simulink model "exampleRadiatorBasic"  (Simulink 7.6)
settings: Solver=ode45  StartTime=0.0  StopTime=8*3600  RelTol=1e-3
undefined symbols (not defined in the file): A, B, C, Dd
libraries: carnot x6
settings Model: Creator=drhf  LastModifiedBy=drhf

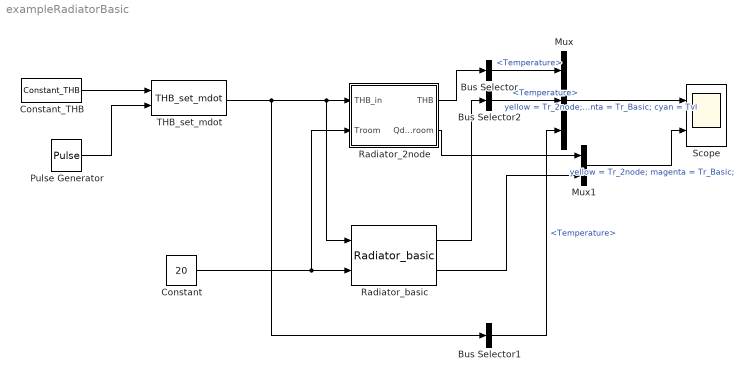
== system exampleRadiatorBasic ==
  Bus Selector : BusSelector  OutputSignals=Temperature
  Bus Selector1 : BusSelector  OutputSignals=Temperature
  Bus Selector2 : BusSelector  OutputSignals=Temperature
  Constant : Constant  Value=20
  Constant_THB : carnot/Source/Simple/Constant_THB  SystemSampleTime=-1  t=75  mdot=0*100/3600  p=1e5  mID=No Pressure Drop  fluid=Water  mix=0  dia=0.02  hgt=0
  Mux : Mux  Inputs=3
  Mux1 : Mux  Inputs=2
  Pulse Generator : DiscretePulseGenerator  PulseType=Time based  Amplitude=100/3600  Period=4*3600  PulseWidth=50
  Radiator_2node : Subsystem  mask(basic radiator){pnom=1200, dtnom=50, expo=1.3, mcp=4182*1, lin=100, qua=100}
      mask prompts: pnom "Qdot_nom: nominal power per in W"; dtnom "Tdiff_nom: nominal temperature difference in K"; expo "radiator exponent (> 0)"; mcp "mass * capacity per unit in J/K"; lin "linear pressure drop"; qua "quadratic pressure drop"
      mask help:
      | The block calculates the heat transfer of a radiator to a room according to the EN 442 equation.
      | A quadratic pressure drop is applied to the fluid flow.
  Radiator_basic : carnot/Basic/Thermal_Models/Radiator_basic  SystemSampleTime=-1  pnomEN=1000  dtnomEN=50  expo=1.3  mcp=4182*1
  Scope : Scope  NumInputPorts=2
      settings: YMin=-5~-5  YMax=5~5
  THB_set_mdot : carnot/Source/Simple/THB_set_mdot  SystemSampleTime=-1
  wires:
  Constant/1 -> Radiator_2node/2(Troom), Radiator_basic/2
  Constant_THB/1 -> THB_set_mdot/1
  THB_set_mdot/1 -> Radiator_2node/1(THB_in), Radiator_basic/1, Bus Selector1/1
  Pulse Generator/1 -> THB_set_mdot/2
  Radiator_2node/1(THB) -> Bus Selector/1
  Bus Selector/1 -> Mux/1  "<Temperature>"
  Mux/1 -> Scope/1  "yellow = Tr_2node; magenta = Tr_Basic; cyan = Tvl"
  Radiator_2node/2(Qdot2room) -> Mux1/1
  Mux1/1 -> Scope/2  "yellow = Tr_2node; magenta = Tr_Basic;"
  Radiator_basic/2 -> Mux1/2
  Radiator_basic/1 -> Bus Selector2/1
  Bus Selector2/1 -> Mux/2  "<Temperature>"
  Bus Selector1/1 -> Mux/3  "<Temperature>"

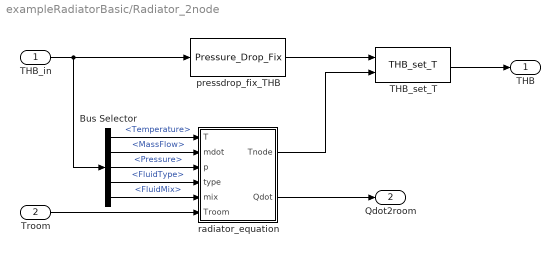
== system exampleRadiatorBasic/Radiator_2node ==
  THB_in : Inport
  Troom : Inport  Port=2
  Bus Selector : BusSelector  OutputSignals=Temperature,MassFlow,Pressure,FluidType,FluidMix
  THB_set_T : carnot/Source/Simple/THB_set_T  SystemSampleTime=-1
  pressdrop_fix_THB : carnot/Basic/Pressure_Drop/Pressure_Drop_Fix  SystemSampleTime=-1  con=0  lin=lin  qua=qua
  radiator_equation : Subsystem  mask(radiator equation){pnom=pnom, dtnom=dtnom, expo=expo, mcap=mcp}
      mask prompts: pnom "Qdot_nom: nominal power per in W"; dtnom "Tdiff_nom: nominal temperature difference in K"; expo "radiator exponent (> 0)"; mcap "mass * capacity per unit in J/K"
      mask help:
      | The block calculates the heat transfer of a radiator to a room according to the EN 442 equation:
      | Qdot = Qdot_nom * (Tdiff/Tdiff_nom)^exponent
      | The thermal capacity of the radiator is modeled by a 1-node capacity.
      | mcp*dT/dt = mdot*cp*(Tin-Tnode)-Qdot
  THB : Outport
  Qdot2room : Outport  Port=2
  wires:
  radiator_equation/2(Qdot) -> Qdot2room/1
  Troom/1 -> radiator_equation/6(Troom)
  radiator_equation/1(Tnode) -> THB_set_T/2
  THB_in/1 -> Bus Selector/1, pressdrop_fix_THB/1
  pressdrop_fix_THB/1 -> THB_set_T/1
  THB_set_T/1 -> THB/1
  Bus Selector/3 -> radiator_equation/3(p)  "<Pressure>"
  Bus Selector/4 -> radiator_equation/4(type)  "<FluidType>"
  Bus Selector/5 -> radiator_equation/5(mix)  "<FluidMix>"
  Bus Selector/2 -> radiator_equation/2(mdot)  "<MassFlow>"
  Bus Selector/1 -> radiator_equation/1(T)  "<Temperature>"

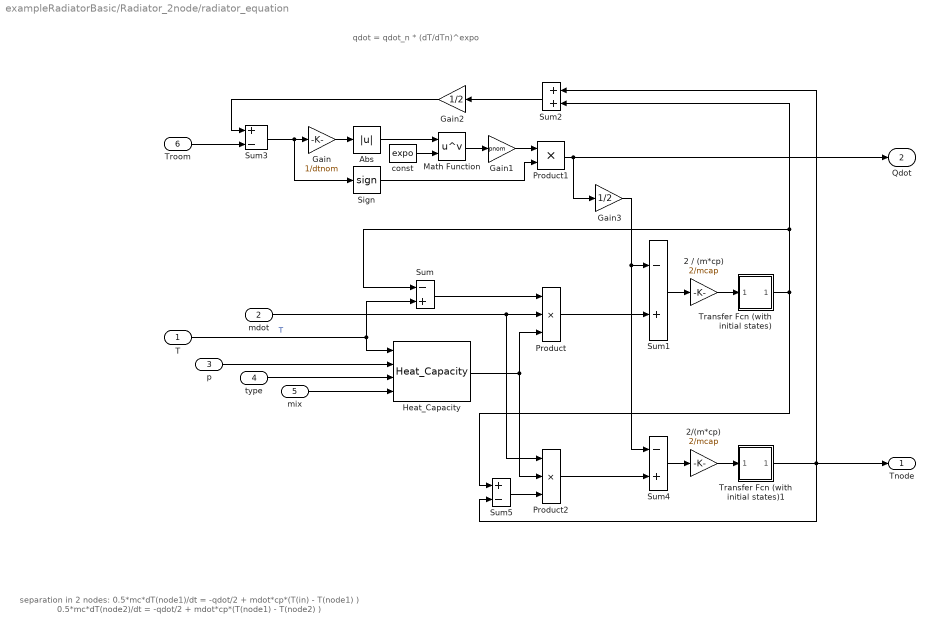
== system exampleRadiatorBasic/Radiator_2node/radiator_equation ==
  note: separation in 2 nodes:
      | 0.5*mc*dT(node1)/dt = -qdot/2 + mdot*cp*(T(in) - T(node1) )
      | 0.5*mc*dT(node2)/dt = -qdot/2 + mdot*cp*(T(node1) - T(node2) )
  note: qdot = qdot_n * (dT/dTn)^expo
  T : Inport
  mdot : Inport  Port=2
  p : Inport  Port=3
  type : Inport  Port=4
  mix : Inport  Port=5
  Troom : Inport  Port=6
  2 / (m*cp) : Gain  Gain=2/mcap  SaturateOnIntegerOverflow=on  OutDataTypeStr=Inherit: Same as input  ParamDataTypeStr=Inherit: Same as input
  2/(m*cp) : Gain  Gain=2/mcap  SaturateOnIntegerOverflow=on  OutDataTypeStr=Inherit: Same as input  ParamDataTypeStr=Inherit: Same as input
  Abs : Abs  SaturateOnIntegerOverflow=on
  Gain : Gain  Gain=1/dtnom  SaturateOnIntegerOverflow=on  OutDataTypeStr=Inherit: Same as input  ParamDataTypeStr=Inherit: Same as input
  Gain1 : Gain  Gain=pnom  SaturateOnIntegerOverflow=on  OutDataTypeStr=Inherit: Same as input  ParamDataTypeStr=Inherit: Same as input
  Gain2 : Gain  Gain=1/2  SaturateOnIntegerOverflow=on  OutDataTypeStr=Inherit: Same as input  ParamDataTypeStr=Inherit: Same as input
  Gain3 : Gain  Gain=1/2  SaturateOnIntegerOverflow=on  OutDataTypeStr=Inherit: Same as input  ParamDataTypeStr=Inherit: Same as input
  Heat_Capacity : carnot/Basic/Material_Properties/Heat_Capacity  SystemSampleTime=-1  VariantObject=CarlibClassic  INPUTARGUMENTS=state variables (classic)  DEBUGLEVEL=DEBUGLEVEL  MAXTOTALWARNINGS=inf  MAXCONSECUTIVEWARNINGS=inf  WRITETOFILE=0  FILENAME='errors.txt'
  Math Function : Math  Operator=pow  SaturateOnIntegerOverflow=on
  Product : Product  Inputs=3  SaturateOnIntegerOverflow=on  InputSameDT=on  OutDataTypeStr=Inherit: Same as first input
  Product1 : Product  SaturateOnIntegerOverflow=on  InputSameDT=on  OutDataTypeStr=Inherit: Same as first input
  Product2 : Product  Inputs=3  SaturateOnIntegerOverflow=on  InputSameDT=on  OutDataTypeStr=Inherit: Same as first input
  Sign : Signum
  Sum : Sum  Inputs=-+  SaturateOnIntegerOverflow=on  InputSameDT=on  OutDataTypeStr=Inherit: Same as first input
  Sum1 : Sum  Inputs=-+  SaturateOnIntegerOverflow=on  InputSameDT=on  OutDataTypeStr=Inherit: Same as first input
  Sum2 : Sum  Inputs=2  SaturateOnIntegerOverflow=on  InputSameDT=on  OutDataTypeStr=Inherit: Same as first input
  Sum3 : Sum  Inputs=+-  SaturateOnIntegerOverflow=on  InputSameDT=on  OutDataTypeStr=Inherit: Same as first input
  Sum4 : Sum  Inputs=-+  SaturateOnIntegerOverflow=on  InputSameDT=on  OutDataTypeStr=Inherit: Same as first input
  Sum5 : Sum  Inputs=+-  SaturateOnIntegerOverflow=on  InputSameDT=on  OutDataTypeStr=Inherit: Same as first input
  Transfer Fcn (with initial states) : Subsystem  mask(Transfer Function with Initial States){N=[1], D=[1  0], X0=20}
      mask prompts: N "Numerator:"; D "Denominator:"; X0 "Initial conditions:"
      mask help: Vector expressions for numerator, and denominator. Coefficients are in descending powers of s.
      mask init:
      | [A,B,C,Dd]=tf2ss(N,D);if (isempty(X0));[m,n]=size(A);X0=zeros(1,m); end;
      mask Help: Specify the initial states for the transfer function.  The state ordering is determined by the m-file tf2ss.  There is no unique mapping of the states in a transfer function to states in a state-space representation.  However, tf2ss will consistently use the same mapping for a given transfer function.
      mask Display: dpoly(N,D,'s')
  Transfer Fcn (with initial states)1 : Subsystem  mask(Transfer Function with Initial States){N=[1], D=[1  0], X0=20}
      mask prompts: N "Numerator:"; D "Denominator:"; X0 "Initial conditions:"
      mask help: Vector expressions for numerator, and denominator. Coefficients are in descending powers of s.
      mask init:
      | [A,B,C,Dd]=tf2ss(N,D);if (isempty(X0));[m,n]=size(A);X0=zeros(1,m); end;
      mask Help: Specify the initial states for the transfer function.  The state ordering is determined by the m-file tf2ss.  There is no unique mapping of the states in a transfer function to states in a state-space representation.  However, tf2ss will consistently use the same mapping for a given transfer function.
      mask Display: dpoly(N,D,'s')
  const : Constant  Value=expo
  Tnode : Outport
  Qdot : Outport  Port=2
  wires:
  Transfer Fcn (with initial states)/1(Out1) -> Sum2/2, Sum/1, Sum5/1
  2 / (m*cp)/1 -> Transfer Fcn (with initial states)/1(In1)
  Sum1/1 -> 2 / (m*cp)/1
  Product/1 -> Sum1/2
  Heat_Capacity/1 -> Product/3, Product2/2
  T/1 -> Sum/2, Heat_Capacity/1  "T"
  mdot/1 -> Product/2, Product2/1
  Sum/1 -> Product/1
  p/1 -> Heat_Capacity/2
  type/1 -> Heat_Capacity/3
  mix/1 -> Heat_Capacity/4
  Product1/1 -> Qdot/1, Gain3/1
  const/1 -> Math Function/2
  Math Function/1 -> Gain1/1
  Gain/1 -> Abs/1
  Abs/1 -> Math Function/1
  Gain1/1 -> Product1/1
  Sum3/1 -> Gain/1, Sign/1
  Sign/1 -> Product1/2
  Troom/1 -> Sum3/2
  Gain2/1 -> Sum3/1
  Sum2/1 -> Gain2/1
  2/(m*cp)/1 -> Transfer Fcn (with initial states)1/1(In1)
  Sum4/1 -> 2/(m*cp)/1
  Gain3/1 -> Sum1/1, Sum4/1
  Sum5/1 -> Product2/3
  Transfer Fcn (with initial states)1/1(Out1) -> Sum5/2, Tnode/1, Sum2/1
  Product2/1 -> Sum4/2

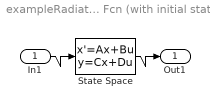
== system exampleRadiatorBasic/Radiator_2node/radiator_equation/Transfer Fcn (with initial states) ==
  In1 : Inport
  State Space : StateSpace  A=A  B=B  C=C  D=Dd  X0=X0
  Out1 : Outport  InitialOutput=0
  wires:
  In1/1 -> State Space/1
  State Space/1 -> Out1/1

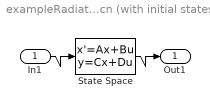
== system exampleRadiatorBasic/Radiator_2node/radiator_equation/Transfer Fcn (with initial states)1 ==
  In1 : Inport
  State Space : StateSpace  A=A  B=B  C=C  D=Dd  X0=X0
  Out1 : Outport  InitialOutput=0
  wires:
  State Space/1 -> Out1/1
  In1/1 -> State Space/1
